simulink model "WCDMA_QPSK"  (R2015a)
settings: Solver=ode45  StartTime=0.0  StopTime=10.0  RelTol=1e-3
undefined symbols (not defined in the file or in its folder): get
libraries: commsrccod2 x2, commdigbbndpm3 x2, commfilt2 x2, commrandsrc2 x1, dspsnks4 x1, commsink2 x1, commseqgen2 x1, dspsigops x1, dspmathops x1
settings Model: Creator=user  LastModifiedBy=user

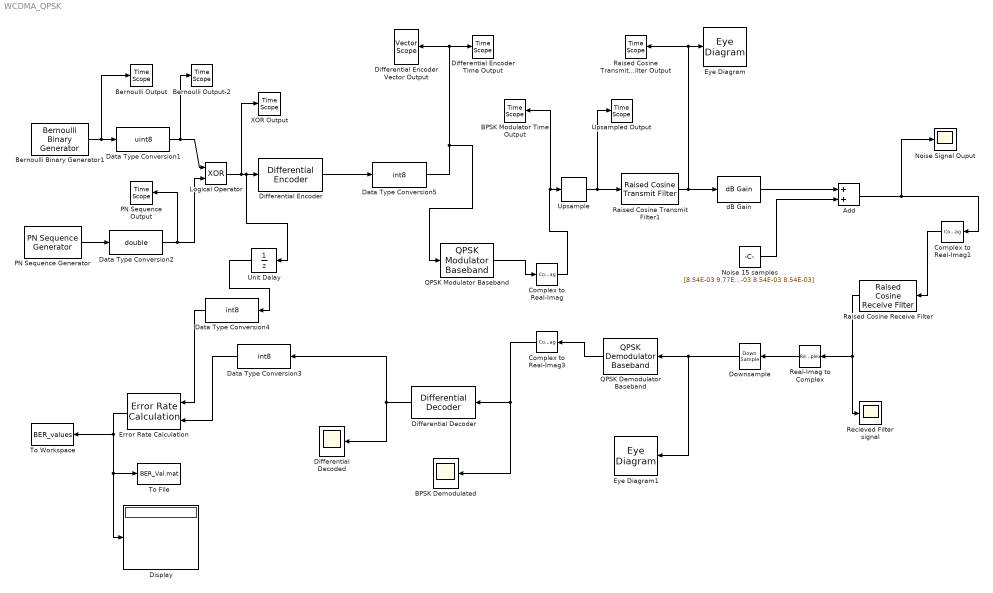
== system WCDMA_QPSK ==
  Add : Sum
  BPSK Demodulated : Scope
      settings: SaveName=ScopeData10
  BPSK Modulator Time Output : TimeScope  DefaultConfigurationName=spbscopes.TimeScopeBlockCfg
  Bernoulli Output : TimeScope  DefaultConfigurationName=spbscopes.TimeScopeBlockCfg
  Bernoulli Output-2 : TimeScope  DefaultConfigurationName=spbscopes.TimeScopeBlockCfg
  Bernoulli Binary Generator1 : commrandsrc2/Bernoulli Binary Generator  P=0.5  seed=61  Ts=1/38400  frameBased=off  sampPerFrame=1  orient=on  outDataType=double
  Complex to Real-Imag : ComplexToRealImag  Output=Real
  Complex to Real-Imag1 : ComplexToRealImag  Output=Real
  Complex to Real-Imag3 : ComplexToRealImag  Output=Real
  Data Type Conversion1 : DataTypeConversion  OutDataTypeStr=uint8
  Data Type Conversion2 : DataTypeConversion  OutDataTypeStr=double
  Data Type Conversion3 : DataTypeConversion  OutDataTypeStr=int8
  Data Type Conversion4 : DataTypeConversion  OutDataTypeStr=int8
  Data Type Conversion5 : DataTypeConversion  OutDataTypeStr=int8
  Differential Decoded : Scope
      settings: SaveName=ScopeData11
  Differential Decoder : commsrccod2/Differential Decoder  InitCond=0
  Differential Encoder : commsrccod2/Differential Encoder  InitCond=0
  Differential Encoder Time Output : TimeScope  DefaultConfigurationName=spbscopes.TimeScopeBlockCfg
  Differential Encoder Vector Output : dspsnks4/Vector Scope  ScopeProperties=on  Domain=Time  HorizSpan=10  DisplayProperties=off  AxisGrid=on  Memory=off  FrameNumber=on  AxisLegend=off  AxisZoom=off  OpenScopeAtSimStart=on  OpenScopeImmediately=off  FigPos=get(0,'defaultfigureposition')  AxisProperties=off  XUnits=Hertz  XRange=[0...Fs/2]  InheritXIncr=on  XIncr=1  XLabel=Time  XLimit=Auto  XMin=0  XMax=1  XStart=0  YUnits=dB  YLabel=Amplitude  LineProperties=off  XAxisParamsVer=6.9
      settings: YMin=-10  YMax=10
  Display : Display
  Downsample : DownSample  N=15  RateOptions=Allow multirate processing
  Error Rate Calculation : commsink2/Error Rate Calculation  N=1  st_delay=0  cp_mode=Entire frame  subframe=[]  PMode=Port  WsName=ErrorVec  RsMode2=off  stop=off  numErr=100  maxBits=1e6
  Eye Diagram : EyeDiagram
  Eye Diagram1 : EyeDiagram
  Logical Operator : Logic  Operator=XOR  AllPortsSameDT=off  OutDataTypeStr=boolean
  Noise Signal Ouput : Scope
      settings: YMin=-4.5  YMax=4.5
  Noise 15 samples : Constant  Value=|
      | [8.54E-03
      | 9.77E-03
      | 8.54E-03
      | 8.54E-03
      | 8.54E-03
      | 8.54E-03
      | 9.77E-03
      | 8.54E-03
      | 8.54E-03
      | 8.54E-03
      | 8.54E-03
      | 8.54E-03
      | 8.54E-03
      | 8.54E-03
      | 8.54E-03]
  PN Sequence Generator : commseqgen2/PN Sequence Generator  poly=[1 0 0 0 0 1 1]  ini_sta=[0 0 0 0 0 1]  outBitMaskSource=Dialog parameter  shift=0  outVarSiz=off  maxOutSizeMode=Dialog parameter  maxOutSize=[10 1]  Ts=1/6400  frameBased=off  sampPerFrame=1  reset=off  bitPackedOutputs=off  outDataType=Smallest unsigned integer  numPackedBits=8  bitPackDataSigned=off  bitPackedOutDType=double
  PN Sequence Output : TimeScope  DefaultConfigurationName=spbscopes.TimeScopeBlockCfg
  QPSK Demodulator Baseband : commdigbbndpm3/QPSK Demodulator Baseband  Ph=pi/4  Dec=Gray  OutType=Integer  DecType=Hard decision  VarSource=Dialog  Variance=1  outDtype1=Inherit via internal rule  outDtype2=Inherit via internal rule  derotateFactorWordLen=16
  QPSK Modulator Baseband : commdigbbndpm3/QPSK Modulator Baseband  InType=Integer  Enc=Gray  Ph=pi/4  outDtype=double  outWordLen=16  outUDDataType=sfix(16)  outFracLenMode=Best precision  outFracLen=15
  Raised Cosine Receive Filter : commfilt2/Raised Cosine Receive Filter  filtType=Square root  N=6  filtSpan=12  currentFiltSpan=12  D=(12)/2  R=0.22  sampMode=Mute  saveAsFlag=0  rateMode=Downsampling  downFactor=1  downOffset=0  framing=Enforce single-rate processing  InputProcessing=Columns as channels (frame based)  checkGain=Normalized  filterGain=1  checkCoeff=off  variableName=rcRxFilt  launchFVT=on  roundingMode=Floor  overflowMode=off
  Raised Cosine Transmit Filter Output : TimeScope  DefaultConfigurationName=spbscopes.TimeScopeBlockCfg
  Raised Cosine Transmit Filter1 : commfilt2/Raised Cosine Transmit Filter  filtType=Square root  filtSpan=12  currentFiltSpan=12  D=(12)/2  R=0.22  sampMode=Mute  saveAsFlag=0  N=6  framing=Allow multirate processing  checkGain=Normalized  filterGain=1  checkCoeff=off  variableName=rcTxFilt1  launchFVT=on  roundingMode=Floor  overflowMode=off
  Real-Imag to Complex : RealImagToComplex  Input=Real
  Recieved Filter signal : Scope
      settings: YMin=-2.25  YMax=2.25  SaveName=ScopeData9
  To File : ToFile  Filename=BER_Val.mat  MatrixName=BER
  To Workspace : ToWorkspace  VariableName=BER_values  SampleTime=-1
  Unit Delay : UnitDelay  SampleTime=1/100
  Upsample : dspsigops/Upsample  N=15  phase=0  InputProcessing=Columns as channels (frame based)  RateOptions=Enforce single-rate processing  ic=0  mode=Unused parameter value
  Upsampled Output : TimeScope  DefaultConfigurationName=spbscopes.TimeScopeBlockCfg
  XOR Output : TimeScope  DefaultConfigurationName=spbscopes.TimeScopeBlockCfg
  dB Gain : dspmathops/dB Gain  dB=5  intype=Amplitude
  wires:
  Bernoulli Binary Generator1/1 -> Bernoulli Output/1, Data Type Conversion1/1
  Data Type Conversion1/1 -> Logical Operator/1, Bernoulli Output-2/1
  PN Sequence Generator/1 -> Data Type Conversion2/1
  Data Type Conversion2/1 -> PN Sequence Output/1, Logical Operator/2
  Logical Operator/1 -> Unit Delay/1, Differential Encoder/1, XOR Output/1
  Differential Encoder/1 -> Data Type Conversion5/1
  Upsample/1 -> Raised Cosine Transmit Filter1/1, Upsampled Output/1
  Raised Cosine Transmit Filter1/1 -> dB Gain/1, Eye Diagram/1, Raised Cosine Transmit Filter Output/1
  dB Gain/1 -> Add/1
  Noise 15 samples/1 -> Add/2
  Add/1 -> Noise Signal Ouput/1, Complex to Real-Imag1/1
  QPSK Modulator Baseband/1 -> Complex to Real-Imag/1
  Complex to Real-Imag/1 -> BPSK Modulator Time Output/1, Upsample/1
  Raised Cosine Receive Filter/1 -> Recieved Filter signal/1, Real-Imag to Complex/1
  Unit Delay/1 -> Data Type Conversion4/1
  Differential Decoder/1 -> Data Type Conversion3/1, Differential Decoded/1
  Data Type Conversion4/1 -> Error Rate Calculation/1
  Error Rate Calculation/1 -> To Workspace/1, Display/1, To File/1
  QPSK Demodulator Baseband/1 -> Complex to Real-Imag3/1
  Downsample/1 -> QPSK Demodulator Baseband/1, Eye Diagram1/1
  Complex to Real-Imag3/1 -> BPSK Demodulated/1, Differential Decoder/1
  Data Type Conversion3/1 -> Error Rate Calculation/2
  Data Type Conversion5/1 -> QPSK Modulator Baseband/1, Differential Encoder Vector Output/1, Differential Encoder Time Output/1
  Complex to Real-Imag1/1 -> Raised Cosine Receive Filter/1
  Real-Imag to Complex/1 -> Downsample/1
